simulink model "ModeloCompletoConTransfereciaVariable"  (R2018a)
settings: Solver=VariableStepAuto  StartTime=0.0  StopTime=10.0  RelTol=1e-3
undefined symbols (not defined in the file): H, k, Kin, m, R
libraries: cstblocks x2
settings Model: Creator=54249  LastModifiedBy=54249

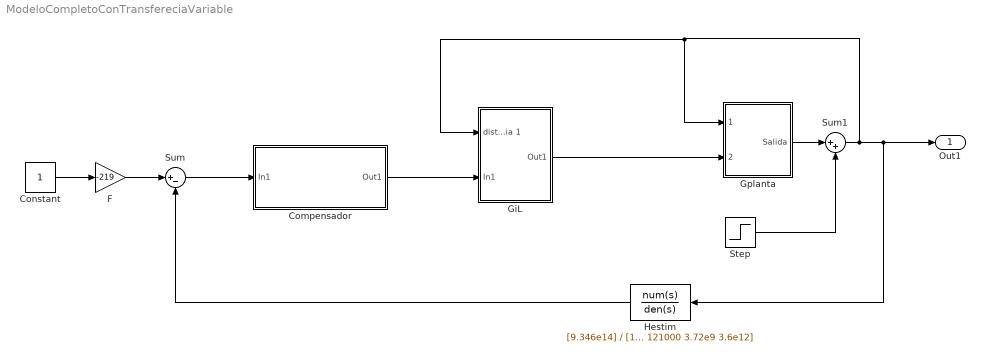
== system ModeloCompletoConTransfereciaVariable ==
  "Compensador " : Subsystem
  Constant : Constant
  "F " : Gain  Gain=-219
  "GiL " : Subsystem
  "Gplanta " : Subsystem
  "Hestim " : TransferFcn  Numerator=[9.346e14]  Denominator=[1 121000 3.72e9 3.6e12]
  Step : Step  Time=0.2  Before=1  After=0  SampleTime=0
  Sum : Sum  Inputs=|+-
  Sum1 : Sum  Inputs=|++
  Out1 : Outport
  wires:
  "Hestim "/1 -> Sum/2
  "F "/1 -> Sum/1
  Sum/1 -> "Compensador "/1(In1)
  "Compensador "/1(Out1) -> "GiL "/2(In1)
  Constant/1 -> "F "/1
  "GiL "/1(Out1) -> "Gplanta "/2(Entrada)
  "Gplanta "/1("Salida ") -> Sum1/1
  Sum1/1 -> "Hestim "/1, Out1/1, "GiL "/1(distancia 1), "Gplanta "/1("distancia ")
  Step/1 -> Sum1/2

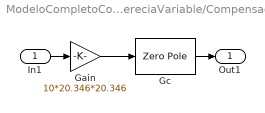
== system ModeloCompletoConTransfereciaVariable/Compensador  ==
  In1 : Inport
  Gain : Gain  Gain=10*20.346*20.346
  Gc : ZeroPole  Zeros=[-44.3 -44.3]  Poles=[-902.1 -902.1]
  Out1 : Outport
  wires:
  Gain/1 -> Gc/1
  Gc/1 -> Out1/1
  In1/1 -> Gain/1

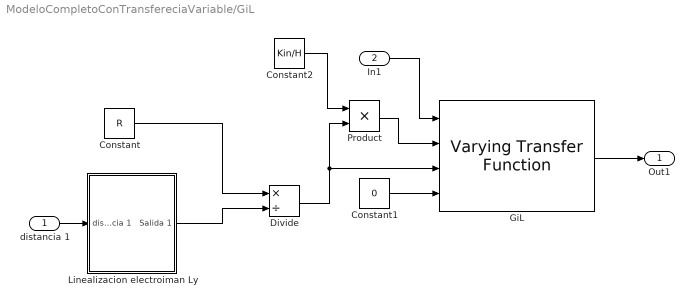
== system ModeloCompletoConTransfereciaVariable/GiL  ==
  distancia 1 : Inport
  In1 : Inport  Port=2
  Constant : Constant  Value=R
  Constant1 : Constant  Value=0
  Constant2 : Constant  Value=Kin/H
  Divide : Product  Inputs=*/
  GiL : cstblocks/Linear Parameter Varying/Varying Transfer Function  N=1
      settings: SourceProductName=Control System Toolbox
  "Linealizacion electroiman Ly " : Subsystem
  Product : Product
  Out1 : Outport
  wires:
  distancia 1/1 -> "Linealizacion electroiman Ly "/1(distancia 1)
  Product/1 -> GiL/2
  Divide/1 -> Product/2, GiL/3
  In1/1 -> GiL/1
  Constant1/1 -> GiL/4
  Constant2/1 -> Product/1
  Constant/1 -> Divide/1
  "Linealizacion electroiman Ly "/1(Salida 1) -> Divide/2
  GiL/1 -> Out1/1

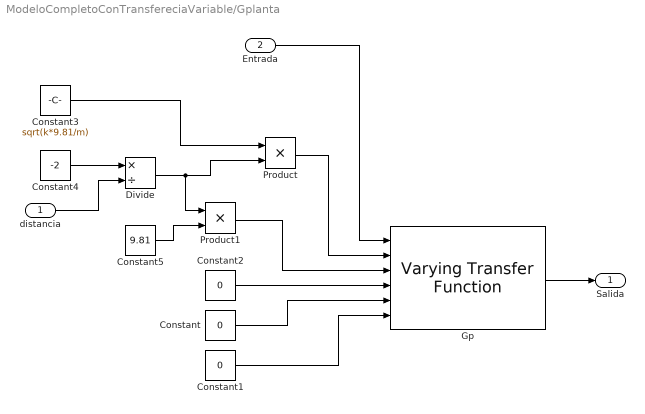
== system ModeloCompletoConTransfereciaVariable/Gplanta  ==
  "distancia " : Inport
  Entrada : Inport  Port=2
  Constant : Constant  Value=0
  Constant1 : Constant  Value=0
  Constant2 : Constant  Value=0
  Constant3 : Constant  Value=sqrt(k*9.81/m)
  Constant4 : Constant  Value=-2
  Constant5 : Constant  Value=9.81
  Divide : Product  Inputs=*/
  Gp : cstblocks/Linear Parameter Varying/Varying Transfer Function  N=2
      settings: SourceProductName=Control System Toolbox
  Product : Product
  Product1 : Product
  "Salida " : Outport
  wires:
  Product1/1 -> Gp/3
  Constant3/1 -> Product/1
  Constant1/1 -> Gp/6
  Divide/1 -> Product1/1, Product/2
  Constant2/1 -> Gp/4
  Gp/1 -> "Salida "/1
  Constant/1 -> Gp/5
  Entrada/1 -> Gp/1
  Constant4/1 -> Divide/1
  Constant5/1 -> Product1/2
  Product/1 -> Gp/2
  "distancia "/1 -> Divide/2

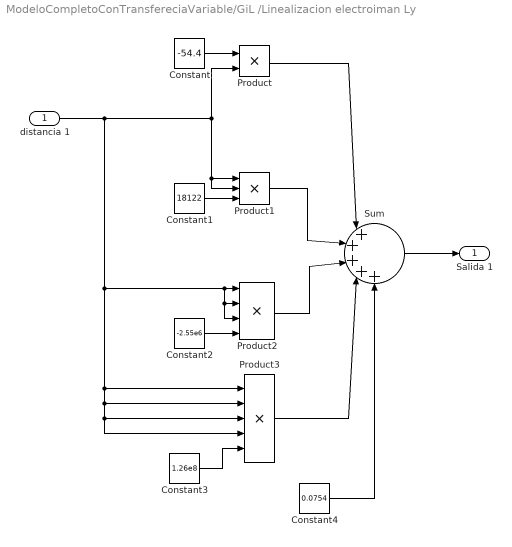
== system ModeloCompletoConTransfereciaVariable/GiL /Linealizacion electroiman Ly  ==
  distancia 1 : Inport
  Constant : Constant  Value=-54.4
  Constant1 : Constant  Value=18122
  Constant2 : Constant  Value=-2.55e6
  Constant3 : Constant  Value=1.26e8
  Constant4 : Constant  Value=0.0754
  Product : Product
  Product1 : Product  Inputs=3
  Product2 : Product  Inputs=4
  Product3 : Product  Inputs=5
  Sum : Sum  Inputs=|+++++
  Salida 1 : Outport
  wires:
  Product1/1 -> Sum/2
  Product3/1 -> Sum/4
  distancia 1/1 -> Product3/1, Product3/2, Product3/3, Product3/4, Product2/1, Product2/2, Product2/3, Product1/1, Product1/2, Product/2
  Constant3/1 -> Product3/5
  Constant/1 -> Product/1
  Product/1 -> Sum/1
  Constant2/1 -> Product2/4
  Constant4/1 -> Sum/5
  Product2/1 -> Sum/3
  Sum/1 -> Salida 1/1
  Constant1/1 -> Product1/3
